simulink model "LKASampleSimulink"  (Simulink 9.1)
settings: Solver=ode1  StartTime=0.0  StopTime=inf  FixedStep=0.001  RelTol=1e-3
InitFcn:
  | load('LKAExampleVariable.mat')
values from neighbouring files (symbols this model uses):
  DataStoreNumPara = 0    [LKAExampleVariable.mat]
  headwayOffset = 3.7    [LKAExampleVariable.mat]
undefined symbols (not defined in the file or in its folder): azimuth_angle, BrStatus, elevation_angle, GroundTruth_Objects, heading, id, Lane_Car_Distance_Left, Lane_Car_Distance_Right, Lane_Class, Lane_Coefficient_C0, Lane_Coefficient_C1, Lane_Coefficient_C2, Lane_Coefficient_C3, Lane_Curvature, Lane_Distance, Lane_ID, LaneInfoPerception, range_bbox, range_center, shape, time, Timestamp, type, velocity, width
libraries: mpcadaslib x1
(part 2 of 2)

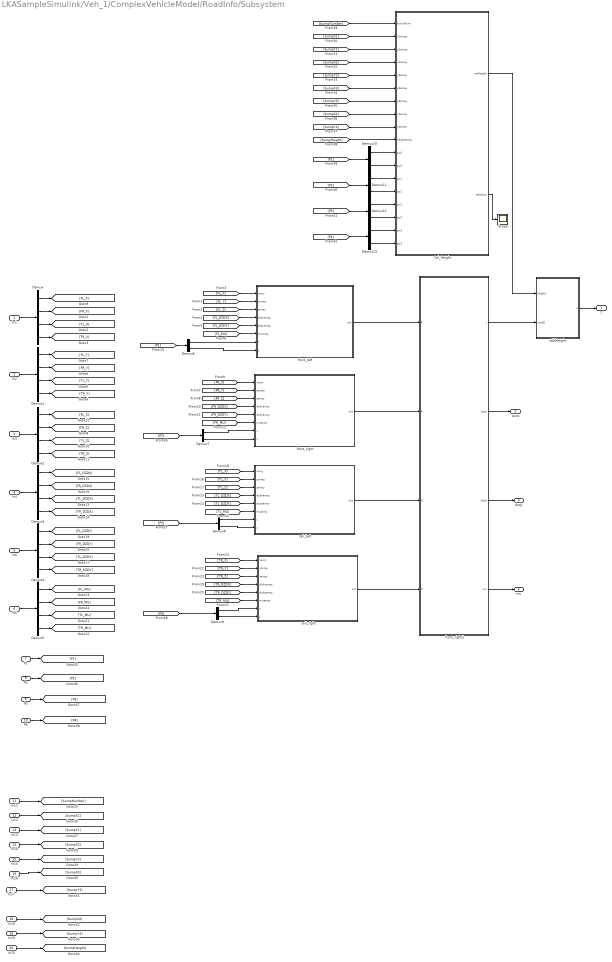
== system LKASampleSimulink/Veh_1/ComplexVehicleModel/RoadInfo/Subsystem ==
  In1 : Inport
  In2 : Inport  Port=2
  In3 : Inport  Port=3
  In4 : Inport  Port=4
  In6 : Inport  Port=5
  In5 : Inport  Port=6
  P1 : Inport  Port=7
  P2 : Inport  Port=8
  P3 : Inport  Port=9
  P4 : Inport  Port=10
  In11 : Inport  Port=11
  In12 : Inport  Port=12
  In13 : Inport  Port=13
  In14 : Inport  Port=14
  In15 : Inport  Port=15
  In16 : Inport  Port=16
  In17 : Inport  Port=17
  In18 : Inport  Port=18
  In19 : Inport  Port=19
  In20 : Inport  Port=20
  AddHeight : MATLAB Function  TreatAsAtomicUnit=on
  Cal_Height : MATLAB Function  TreatAsAtomicUnit=on
  Demux{,1..5} (6 alike) : Demux
  Demux{6..13} (8 alike) : Demux  Outputs=2
  Scope : Scope
  front_left : MATLAB Function  TreatAsAtomicUnit=on
  front_right : MATLAB Function  TreatAsAtomicUnit=on
  front_right1 : MATLAB Function  TreatAsAtomicUnit=on
  tail_left : MATLAB Function  TreatAsAtomicUnit=on
  tail_right : MATLAB Function  TreatAsAtomicUnit=on
  z : Outport  VectorParamsAs1DForOutWhenUnconnected=off
  dzdx : Outport  Port=2  VectorParamsAs1DForOutWhenUnconnected=off
  dzdy : Outport  Port=3  VectorParamsAs1DForOutWhenUnconnected=off
  mu : Outport  Port=4  VectorParamsAs1DForOutWhenUnconnected=off
  wires:
  Cal_Height/2(retValue) -> Scope/1
  AddHeight/1(z) -> z/1
  Cal_Height/1(retHeight) -> AddHeight/1(height)
  [bumpY3] -> Cal_Height/7(y3array)
  Demux11/1 -> Cal_Height/13(px1)
  [bumpHeight] -> Cal_Height/10(heightarray)
  [bumpX1] -> Cal_Height/2(x1array)
  Demux11/2 -> Cal_Height/14(py1)
  [bumpY1] -> Cal_Height/3(y1array)
  [P2] -> Demux11/1
  Demux10/1 -> Cal_Height/11(px0)
  [bumpX3] -> Cal_Height/6(x3array)
  [P3] -> Demux12/1
  Demux10/2 -> Cal_Height/12(py0)
  [bumpNumber] -> Cal_Height/1(bumsNum)
  Demux12/1 -> Cal_Height/15(px2)
  [P4] -> Demux13/1
  Demux12/2 -> Cal_Height/16(py2)
  [bumpY4] -> Cal_Height/9(y4array)
  [bumpX4] -> Cal_Height/8(x4array)
  [P1] -> Demux10/1
  [bumpX2] -> Cal_Height/4(x2array)
  Demux13/1 -> Cal_Height/17(px3)
  Demux13/2 -> Cal_Height/18(py3)
  [bumpY2] -> Cal_Height/5(y2array)
  [P4] -> Demux9/1
  [P3] -> Demux8/1
  [P2] -> Demux7/1
  [P1] -> Demux6/1
  In20/1 -> [bumpHeight]
  In19/1 -> [bumpY4]
  In18/1 -> [bumpX4]
  In17/1 -> [bumpY3]
  In16/1 -> [bumpX3]
  In15/1 -> [bumpY2]
  In14/1 -> [bumpX2]
  In13/1 -> [bumpY1]
  In12/1 -> [bumpX1]
  In11/1 -> [bumpNumber]
  In1/1 -> Demux/1
  Demux/1 -> [FL_X]
  Demux/2 -> [FR_X]
  Demux/3 -> [TL_X]
  Demux/4 -> [TR_X]
  Demux1/1 -> [FL_Y]
  Demux1/3 -> [TL_Y]
  Demux1/4 -> [TR_Y]
  Demux1/2 -> [FR_Y]
  In2/1 -> Demux1/1
  In3/1 -> Demux2/1
  Demux2/4 -> [TR_Z]
  Demux2/3 -> [TL_Z]
  Demux2/2 -> [FR_Z]
  Demux2/1 -> [FL_Z]
  Demux3/4 -> [TR_DZDX]
  In4/1 -> Demux3/1
  Demux3/3 -> [TL_DZDX]
  Demux3/1 -> [FL_DZDX]
  Demux3/2 -> [FR_DZDX]
  Demux4/2 -> [FR_DZDY]
  Demux4/4 -> [TR_DZDY]
  Demux4/1 -> [FL_DZDY]
  Demux4/3 -> [TL_DZDY]
  In6/1 -> Demux4/1
  Demux5/3 -> [TL_MU]
  Demux5/4 -> [TR_MU]
  Demux5/2 -> [FR_MU]
  Demux5/1 -> [FL_MU]
  In5/1 -> Demux5/1
  [FL_X] -> front_left/1(xarry)
  [FL_Y] -> front_left/2(yarray)
  [FL_MU] -> front_left/6(muarray)
  [FL_DZDY] -> front_left/5(dzdyarray)
  [FL_DZDX] -> front_left/4(dzdxarray)
  [FL_Z] -> front_left/3(zarray)
  [FR_X] -> front_right/1(xarry)
  [FR_Y] -> front_right/2(yarray)
  [FR_Z] -> front_right/3(zarray)
  [FR_DZDX] -> front_right/4(dzdxarray)
  [FR_DZDY] -> front_right/5(dzdyarray)
  [FR_MU] -> front_right/6(muarray)
  [TL_X] -> tail_left/1(xarry)
  [TL_Y] -> tail_left/2(yarray)
  [TL_Z] -> tail_left/3(zarray)
  [TL_DZDX] -> tail_left/4(dzdxarray)
  [TL_DZDY] -> tail_left/5(dzdyarray)
  [TL_MU] -> tail_left/6(muarray)
  [TR_X] -> tail_right/1(xarry)
  [TR_Y] -> tail_right/2(yarray)
  [TR_Z] -> tail_right/3(zarray)
  [TR_DZDX] -> tail_right/4(dzdxarray)
  [TR_DZDY] -> tail_right/5(dzdyarray)
  [TR_MU] -> tail_right/6(muarray)
  front_left/1(out) -> front_right1/1(fl)
  front_right/1(out) -> front_right1/2(fr)
  front_right1/1(z) -> AddHeight/2(roadZ)
  front_right1/2(dzdx) -> dzdx/1
  front_right1/3(dzdy) -> dzdy/1
  front_right1/4(mu) -> mu/1
  tail_left/1(out) -> front_right1/3(tl)
  tail_right/1(out) -> front_right1/4(tr)
  P1/1 -> [P1]
  Demux6/1 -> front_left/7(x)
  Demux6/2 -> front_left/8(y)
  P2/1 -> [P2]
  Demux7/1 -> front_right/7(x)
  Demux7/2 -> front_right/8(y)
  Demux8/1 -> tail_left/7(x)
  Demux8/2 -> tail_left/8(y)
  P3/1 -> [P3]
  Demux9/1 -> tail_right/7(x)
  Demux9/2 -> tail_right/8(y)
  P4/1 -> [P4]

== system LKASampleSimulink/Veh_1/ComplexVehicleModel/RoadInfo/Subsystem1 ==
  Rx_eo2ctc_coE_Refine : Inport
  Ry_eo2ctc_coE_Refine : Inport  Port=2
  front_right : MATLAB Function  TreatAsAtomicUnit=on
  P1 : Outport  VectorParamsAs1DForOutWhenUnconnected=off
  P2 : Outport  Port=2  VectorParamsAs1DForOutWhenUnconnected=off
  P3 : Outport  Port=3  VectorParamsAs1DForOutWhenUnconnected=off
  P4 : Outport  Port=4  VectorParamsAs1DForOutWhenUnconnected=off
  wires:
  Rx_eo2ctc_coE_Refine/1 -> front_right/1(array1)
  Ry_eo2ctc_coE_Refine/1 -> front_right/2(array2)
  front_right/2(p2) -> P2/1
  front_right/1(p1) -> P1/1
  front_right/3(p3) -> P3/1
  front_right/4(p4) -> P4/1

== system LKASampleSimulink/Veh_1/VehicleDataBus/GlobalVariableWrite/GlobalVariableSwitch ==
  value : Inport
  time : Inport  Port=2
  originalValue : Inport  Port=3
  originalTime : Inport  Port=4
  GlobalVariable0 : S-Function  FunctionName=BusWriter  Parameters='global.0','time@i,variable@d','0.01','0.0'  SFunctionDeploymentMode=off  EnableBusSupport=off
  Minus : Sum  Inputs=+-
  Switch : Switch  Criteria=u2 ~= 0  Threshold=1
  wires:
  Switch/1 -> GlobalVariable0/1
  originalTime/1 -> Switch/3
  time/1 -> Switch/1
  Minus/1 -> Switch/2
  originalValue/1 -> Minus/2
  value/1 -> Minus/1, GlobalVariable0/2

== system LKASampleSimulink/Veh_1/VehicleDataBus/GlobalVariableWrite/GlobalVariableSwitch1 ==
  value : Inport
  time : Inport  Port=2
  originalValue : Inport  Port=3
  originalTime : Inport  Port=4
  GlobalVariable1 : S-Function  FunctionName=BusWriter  Parameters='global.1','time@i,variable@d','0.01','0.0'  SFunctionDeploymentMode=off  EnableBusSupport=off
  Minus : Sum  Inputs=+-
  Switch : Switch  Criteria=u2 ~= 0  Threshold=1
  wires:
  Switch/1 -> GlobalVariable1/1
  originalTime/1 -> Switch/3
  time/1 -> Switch/1
  Minus/1 -> Switch/2
  originalValue/1 -> Minus/2
  value/1 -> Minus/1, GlobalVariable1/2

== system LKASampleSimulink/Veh_1/VehicleDataBus/GlobalVariableWrite/GlobalVariableSwitch2 ==
  value : Inport
  time : Inport  Port=2
  originalValue : Inport  Port=3
  originalTime : Inport  Port=4
  GlobalVariable2 : S-Function  FunctionName=BusWriter  Parameters='global.2','time@i,variable@d','0.01','0.0'  SFunctionDeploymentMode=off  EnableBusSupport=off
  Minus : Sum  Inputs=+-
  Switch : Switch  Criteria=u2 ~= 0  Threshold=1
  wires:
  Switch/1 -> GlobalVariable2/1
  originalTime/1 -> Switch/3
  time/1 -> Switch/1
  Minus/1 -> Switch/2
  originalValue/1 -> Minus/2
  value/1 -> Minus/1, GlobalVariable2/2

== system LKASampleSimulink/Veh_1/VehicleDataBus/GlobalVariableWrite/GlobalVariableSwitch3 ==
  value : Inport
  time : Inport  Port=2
  originalValue : Inport  Port=3
  originalTime : Inport  Port=4
  GlobalVariable3 : S-Function  FunctionName=BusWriter  Parameters='global.3','time@i,variable@d','0.01','0.0'  SFunctionDeploymentMode=off  EnableBusSupport=off
  Minus : Sum  Inputs=+-
  Switch : Switch  Criteria=u2 ~= 0  Threshold=1
  wires:
  Switch/1 -> GlobalVariable3/1
  originalTime/1 -> Switch/3
  time/1 -> Switch/1
  Minus/1 -> Switch/2
  originalValue/1 -> Minus/2
  value/1 -> Minus/1, GlobalVariable3/2

== system LKASampleSimulink/Veh_1/VehicleDataBus/GlobalVariableWrite/GlobalVariableSwitch4 ==
  value : Inport
  time : Inport  Port=2
  originalValue : Inport  Port=3
  originalTime : Inport  Port=4
  GlobalVariable4 : S-Function  FunctionName=BusWriter  Parameters='global.4','time@i,variable@d','0.01','0.0'  SFunctionDeploymentMode=off  EnableBusSupport=off
  Minus : Sum  Inputs=+-
  Switch : Switch  Criteria=u2 ~= 0  Threshold=1
  wires:
  Switch/1 -> GlobalVariable4/1
  originalTime/1 -> Switch/3
  time/1 -> Switch/1
  Minus/1 -> Switch/2
  originalValue/1 -> Minus/2
  value/1 -> Minus/1, GlobalVariable4/2

== system LKASampleSimulink/Veh_1/VehicleDataBus/GlobalVariableWrite/GlobalVariableSwitch5 ==
  value : Inport
  time : Inport  Port=2
  originalValue : Inport  Port=3
  originalTime : Inport  Port=4
  GlobalVariable5 : S-Function  FunctionName=BusWriter  Parameters='global.5','time@i,variable@d','0.01','0.0'  SFunctionDeploymentMode=off  EnableBusSupport=off
  Minus : Sum  Inputs=+-
  Switch : Switch  Criteria=u2 ~= 0  Threshold=1
  wires:
  Switch/1 -> GlobalVariable5/1
  originalTime/1 -> Switch/3
  time/1 -> Switch/1
  Minus/1 -> Switch/2
  originalValue/1 -> Minus/2
  value/1 -> Minus/1, GlobalVariable5/2

== system LKASampleSimulink/Veh_1/VehicleDataBus/GlobalVariableWrite/GlobalVariableSwitch6 ==
  value : Inport
  time : Inport  Port=2
  originalValue : Inport  Port=3
  originalTime : Inport  Port=4
  GlobalVariable6 : S-Function  FunctionName=BusWriter  Parameters='global.6','time@i,variable@d','0.01','0.0'  SFunctionDeploymentMode=off  EnableBusSupport=off
  Minus : Sum  Inputs=+-
  Switch : Switch  Criteria=u2 ~= 0  Threshold=1
  wires:
  Switch/1 -> GlobalVariable6/1
  originalTime/1 -> Switch/3
  time/1 -> Switch/1
  Minus/1 -> Switch/2
  originalValue/1 -> Minus/2
  value/1 -> Minus/1, GlobalVariable6/2

== system LKASampleSimulink/Veh_1/VehicleDataBus/GlobalVariableWrite/GlobalVariableSwitch7 ==
  value : Inport
  time : Inport  Port=2
  originalValue : Inport  Port=3
  originalTime : Inport  Port=4
  GlobalVariable7 : S-Function  FunctionName=BusWriter  Parameters='global.7','time@i,variable@d','0.01','0.0'  SFunctionDeploymentMode=off  EnableBusSupport=off
  Minus : Sum  Inputs=+-
  Switch : Switch  Criteria=u2 ~= 0  Threshold=1
  wires:
  Switch/1 -> GlobalVariable7/1
  originalTime/1 -> Switch/3
  time/1 -> Switch/1
  Minus/1 -> Switch/2
  originalValue/1 -> Minus/2
  value/1 -> Minus/1, GlobalVariable7/2

== system LKASampleSimulink/Veh_1/VehicleDataBus/GlobalVariableWrite/GlobalVariableSwitch8 ==
  value : Inport
  time : Inport  Port=2
  originalValue : Inport  Port=3
  originalTime : Inport  Port=4
  GlobalVariable8 : S-Function  FunctionName=BusWriter  Parameters='global.8','time@i,variable@d','0.01','0.0'  SFunctionDeploymentMode=off  EnableBusSupport=off
  Minus : Sum  Inputs=+-
  Switch : Switch  Criteria=u2 ~= 0  Threshold=1
  wires:
  Switch/1 -> GlobalVariable8/1
  originalTime/1 -> Switch/3
  time/1 -> Switch/1
  Minus/1 -> Switch/2
  originalValue/1 -> Minus/2
  value/1 -> Minus/1, GlobalVariable8/2

== system LKASampleSimulink/Veh_1/VehicleDataBus/GlobalVariableWrite/GlobalVariableSwitch9 ==
  value : Inport
  time : Inport  Port=2
  originalValue : Inport  Port=3
  originalTime : Inport  Port=4
  GlobalVariable9 : S-Function  FunctionName=BusWriter  Parameters='global.9','time@i,variable@d','0.01','0.0'  SFunctionDeploymentMode=off  EnableBusSupport=off
  Minus : Sum  Inputs=+-
  Switch : Switch  Criteria=u2 ~= 0  Threshold=1
  wires:
  Switch/1 -> GlobalVariable9/1
  originalTime/1 -> Switch/3
  time/1 -> Switch/1
  Minus/1 -> Switch/2
  originalValue/1 -> Minus/2
  value/1 -> Minus/1, GlobalVariable9/2

== system LKASampleSimulink/Veh_1/Algorithm/lane Following Controller/MPC Controller/InValueLimiters ==
  RelativeDistanceIn : Inport
  RelativeVelocityIn : Inport  Port=2
  LongitudinalVelocityIn : Inport  Port=3
  Constant1 : Constant  Value=200
  Constant2 : Constant  Value=0
  Saturation : Saturate  UpperLimit=100  LowerLimit=0.00001
  Switch1 : Switch  Criteria=u2 > Threshold  Threshold=1000
  Switch2 : Switch  Criteria=u2 > Threshold  Threshold=1000
  Relative distance : Outport
  Relative velocity : Outport  Port=2
  Longitudinal velocity : Outport  Port=3
  wires:
  RelativeVelocityIn/1 -> Switch2/3
  Constant2/1 -> Switch2/1
  Constant1/1 -> Switch1/1
  LongitudinalVelocityIn/1 -> Saturation/1
  RelativeDistanceIn/1 -> Switch1/2, Switch1/3, Switch2/2
  Switch2/1 -> Relative velocity/1
  Switch1/1 -> Relative distance/1
  Saturation/1 -> Longitudinal velocity/1

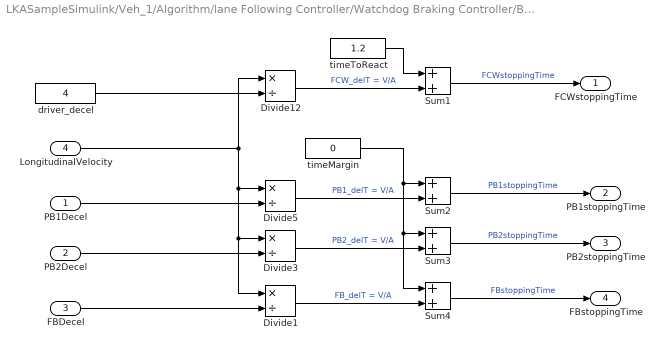
== system LKASampleSimulink/Veh_1/Algorithm/lane Following Controller/Watchdog Braking Controller/BrakeTimeCalculation ==
  PB1Decel : Inport
  PB2Decel : Inport  Port=2
  FBDecel : Inport  Port=3
  LongitudinalVelocity : Inport  Port=4
  Divide{1,3,5,12} (4 alike) : Product  Inputs=*/
  Sum{1..4} (4 alike) : Sum
  driver_decel : Constant  Value=4
  timeMargin : Constant  Value=0
  timeToReact : Constant  Value=1.2
  FCWstoppingTime : Outport
  PB1stoppingTime : Outport  Port=2
  PB2stoppingTime : Outport  Port=3
  FBstoppingTime : Outport  Port=4
  wires:
  Sum2/1 -> PB1stoppingTime/1  "PB1stoppingTime"
  timeMargin/1 -> Sum3/1, Sum4/1, Sum2/1
  Divide12/1 -> Sum1/2  "FCW_delT = V/A"
  LongitudinalVelocity/1 -> Divide3/1, Divide1/1, Divide5/1, Divide12/1
  PB2Decel/1 -> Divide3/2
  Divide1/1 -> Sum4/2  "FB_delT = V/A"
  Divide3/1 -> Sum3/2  "PB2_delT = V/A"
  Divide5/1 -> Sum2/2  "PB1_delT = V/A"
  timeToReact/1 -> Sum1/1
  FBDecel/1 -> Divide1/2
  driver_decel/1 -> Divide12/2
  PB1Decel/1 -> Divide5/2
  Sum4/1 -> FBstoppingTime/1  "FBstoppingTime"
  Sum3/1 -> PB2stoppingTime/1  "PB2stoppingTime"
  Sum1/1 -> FCWstoppingTime/1  "FCWstoppingTime"

== system LKASampleSimulink/Veh_1/Algorithm/lane Following Controller/Watchdog Braking Controller/BrakingLogic ==
  note: Input: relativeDistance, TTC, FCWtime, PB1time, PB2time, FBtime, longVelocity
      | Description: as time to collision gets shorter, request deceleration and signal the braking status. 4 Levels are identified warning, partial braking 1/2 and full braking.
      | Output: BrakeStatus, decel
  relativeDistance : Inport
  TTC : Inport  Port=2
  FCWtime : Inport  Port=3
  PB1time : Inport  Port=4
  PB2time : Inport  Port=5
  FBtime : Inport  Port=6
  longVelocity : Inport  Port=7
  BrakingLogic : Stateflow chart  TreatAsAtomicUnit=on
  RelationalOperator : RelationalOperator  Operator=<=  RndMeth=Simplest
  stopVelThreshold : Constant  Value=0.1
  BrakeStatus : Outport
  decel : Outport  Port=2
  wires:
  RelationalOperator/1 -> BrakingLogic/7(stop)
  relativeDistance/1 -> BrakingLogic/1(relativeDistance)
  BrakingLogic/2(decel) -> decel/1
  TTC/1 -> BrakingLogic/2(TTC)
  PB1time/1 -> BrakingLogic/4(PB1time)
  longVelocity/1 -> RelationalOperator/1
  FBtime/1 -> BrakingLogic/6(FBtime)
  FCWtime/1 -> BrakingLogic/3(FCWtime)
  BrakingLogic/1(BrakeStatus) -> BrakeStatus/1
  PB2time/1 -> BrakingLogic/5(PB2time)
  stopVelThreshold/1 -> RelationalOperator/2

== system LKASampleSimulink/Veh_1/Algorithm/lane Following Controller/Watchdog Braking Controller/TTCCalculation ==
  mioDistance : Inport
  mioVelocity : Inport  Port=2
  Abs : Abs
  Divide11 : Product  Inputs=**
  Divide3 : Product  Inputs=*/
  Saturation : Saturate  UpperLimit=100  LowerLimit=0.01
  Sign : Signum
  Sum : Sum  Inputs=+-
  const1 : Constant  Value=headwayOffset  SampleTime=-1
  TTC : Outport  VectorParamsAs1DForOutWhenUnconnected=off
  wires:
  mioVelocity/1 -> Sign/1, Abs/1
  mioDistance/1 -> Sum/1
  Divide3/1 -> Divide11/1  "TTC"
  const1/1 -> Sum/2
  Sum/1 -> Divide3/1  "headway"
  Abs/1 -> Saturation/1
  Saturation/1 -> Divide3/2
  Sign/1 -> Divide11/2
  Divide11/1 -> TTC/1

== matlab function Veh_1/ComplexVehicleModel/RoadInfo/Subsystem/front_right ==
  data: out output double; xarry input double; yarray input double; zarray input double; dzdxarray input double; dzdyarray input double; muarray input double; x input double; y input double
function out  = fcn(xarry,yarray,zarray,dzdxarray,dzdyarray,muarray,x,y)
[x1,y1,x2,y2,x3,y3,x4,y4] = fcn_getpoint(xarry,yarray);
data_array = fcn_getdata(zarray,dzdxarray, dzdyarray,muarray);

zero = 0.001;
if ( abs(y2-y1) > zero )
   angle = 2*pi -  atan2(y2-y1,x2-x1);
   sin_angle = sin(angle);
   cos_angle = cos(angle);
   [x1,y1] = fcn_convert(x1,y1,x1,y1,sin_angle,cos_angle);
   [x2,y2] = fcn_convert(x1,y1,x2,y2,sin_angle,cos_angle);
   [x3,y3] = fcn_convert(x1,y1,x3,y3,sin_angle,cos_angle);
   [x4,y4] = fcn_convert(x1,y1,x4,y4,sin_angle,cos_angle);
   [x,y] = fcn_convert(x1,y1,x,y,sin_angle,cos_angle);
end

axle_x_left  = min(x1,x2);
axle_x_right = max(x1,x2);
axle_y_up    = max(y2,y3);
axle_y_down  = min(y2,y3);

% after rotota
% p1  p2
%
% p3 p4
z = 0;
dzdx = 0;
dzdy = 0;
mu = 0;
if ( x > axle_x_left ) && ( x < axle_x_right ) && ( y > axle_y_down ) && ( y < axle_y_up )
    xx1 = x3;
    xx2 = x4;
    yy1 = y3;
    yy2 = y1;
    matrix_left = [xx2-x  x-xx1];
    matrix_right = [ yy2 - y; y-yy1 ];
    delta = (xx2-xx1)*(yy2-yy1);
    delta = 1.0/delta;
    [z, dzdx, dzdy, mu] = fcn_cal(matrix_left,matrix_right,delta,data_array);
else
    if ( y >= axle_y_up ) 
        [z, dzdx, dzdy, mu] = fcn_cal_getmax(data_array(1,:),data_array(2,:));
    end
    if ( y <= axle_y_down )
        [z, dzdx, dzdy, mu] = fcn_cal_getmax(data_array(3,:),data_array(4,:));
    end
    if ( x >= axle_x_right )
        [z, dzdx, dzdy, mu] = fcn_cal_getmax(data_array(2,:),data_array(4,:));
    end
    if ( x <= axle_x_left )
        [z, dzdx, dzdy, mu] = fcn_cal_getmax(data_array(1,:),data_array(3,:));
    end
end

out = [z dzdx dzdy mu];
end

function [xxx,yyy] = fcn_convert(x0,y0,x1,y1,sin_agnle,cos_angle)
    xxx = (x1-x0)*cos_angle - (y1-y0)*sin_agnle + x0;
    yyy = (x1-x0)*sin_agnle + (y1-y0)*cos_angle + y0;
end

function [x1,y1,x2,y2,x3,y3,x4,y4] = fcn_getpoint(xarry,yarray)
    x1 = xarry(1);
    x2 = xarry(2);
    x3 = xarry(3);
    x4 = xarry(4);
    y1 = yarray(1);
    y2 = yarray(2);
    y3 = yarray(3);
    y4 = yarray(4);
end

function ret = fcn_getdata(zarray,dzdxarray, dzdyarray,muarray)
    ret = [ 
        zarray(1),dzdxarray(1),dzdyarray(1),muarray(1);
        zarray(2),dzdxarray(2),dzdyarray(2),muarray(2);
        zarray(3),dzdxarray(3),dzdyarray(3),muarray(3);
        zarray(4),dzdxarray(4),dzdyarray(4),muarray(4);
    ];
end

function [z,dzdx,dzdy,mu] = fcn_cal(matrix_left,matrix_right , delta, data_array)
%matrix_z = [z3, z1; z4 , z2]
%value = [xx2-x  x-xx1] * matrix * [ yy2 - y; y-yy1 ]  * d1
    array_z = data_array(:,1);
    array_dzdx = data_array(:,2);
    array_dzdy = data_array(:,3);
    array_mu = data_array(:,4);
    z = matrix_left * [array_z(3), array_z(1); array_z(4),array_z(2)] * matrix_right  * delta;
    dzdx = matrix_left * [array_dzdx(3), array_dzdx(1); array_dzdx(4),array_dzdx(2)] * matrix_right  * delta;
    dzdy = matrix_left * [array_dzdy(3), array_dzdy(1); array_dzdy(4),array_dzdy(2)] * matrix_right  * delta;
    mu = matrix_left * [array_mu(3), array_mu(1); array_mu(4),array_mu(2)] * matrix_right  * delta;
end

function [z,dzdx,dzdy,mu] = fcn_cal_getmax(data1,data2)
    z = max(data1(1),data2(1));
    dzdx = max(data1(2),data2(2));
    dzdy = max(data1(3),data2(3));
    mu = max(data1(4),data2(4));
end

== matlab function Veh_1/ComplexVehicleModel/RoadInfo/Subsystem/front_left ==
  data: out output double; xarry input double; yarray input double; zarray input double; dzdxarray input double; dzdyarray input double; muarray input double; x input double; y input double
function out  = fcn(xarry,yarray,zarray,dzdxarray,dzdyarray,muarray,x,y)
[x1,y1,x2,y2,x3,y3,x4,y4] = fcn_getpoint(xarry,yarray);
data_array = fcn_getdata(zarray,dzdxarray, dzdyarray,muarray);

zero = 0.001;
if ( abs(y2-y1) > zero )
   angle = 2*pi -  atan2(y2-y1,x2-x1);
   sin_angle = sin(angle);
   cos_angle = cos(angle);
   [x1,y1] = fcn_convert(x1,y1,x1,y1,sin_angle,cos_angle);
   [x2,y2] = fcn_convert(x1,y1,x2,y2,sin_angle,cos_angle);
   [x3,y3] = fcn_convert(x1,y1,x3,y3,sin_angle,cos_angle);
   [x4,y4] = fcn_convert(x1,y1,x4,y4,sin_angle,cos_angle);
   [x,y] = fcn_convert(x1,y1,x,y,sin_angle,cos_angle);
end

axle_x_left  = min(x1,x2);
axle_x_right = max(x1,x2);
axle_y_up    = max(y2,y3);
axle_y_down  = min(y2,y3);

% after rotota
% p1  p2
%
% p3 p4
z = 0;
dzdx = 0;
dzdy = 0;
mu = 0;
if ( x > axle_x_left ) && ( x < axle_x_right ) && ( y > axle_y_down ) && ( y < axle_y_up )
    xx1 = x3;
    xx2 = x4;
    yy1 = y3;
    yy2 = y1;
    matrix_left = [xx2-x  x-xx1];
    matrix_right = [ yy2 - y; y-yy1 ];
    delta = (xx2-xx1)*(yy2-yy1);
    delta = 1.0/delta;
    [z, dzdx, dzdy, mu] = fcn_cal(matrix_left,matrix_right,delta,data_array);
else
    if ( y >= axle_y_up ) 
        [z, dzdx, dzdy, mu] = fcn_cal_getmax(data_array(1,:),data_array(2,:));
    end
    if ( y <= axle_y_down )
        [z, dzdx, dzdy, mu] = fcn_cal_getmax(data_array(3,:),data_array(4,:));
    end
    if ( x >= axle_x_right )
        [z, dzdx, dzdy, mu] = fcn_cal_getmax(data_array(2,:),data_array(4,:));
    end
    if ( x <= axle_x_left )
        [z, dzdx, dzdy, mu] = fcn_cal_getmax(data_array(1,:),data_array(3,:));
    end
end

out = [z dzdx dzdy mu];
end

function [xxx,yyy] = fcn_convert(x0,y0,x1,y1,sin_agnle,cos_angle)
    xxx = (x1-x0)*cos_angle - (y1-y0)*sin_agnle + x0;
    yyy = (x1-x0)*sin_agnle + (y1-y0)*cos_angle + y0;
end

function [x1,y1,x2,y2,x3,y3,x4,y4] = fcn_getpoint(xarry,yarray)
    x1 = xarry(1);
    x2 = xarry(2);
    x3 = xarry(3);
    x4 = xarry(4);
    y1 = yarray(1);
    y2 = yarray(2);
    y3 = yarray(3);
    y4 = yarray(4);
end

function ret = fcn_getdata(zarray,dzdxarray, dzdyarray,muarray)
    ret = [ 
        zarray(1),dzdxarray(1),dzdyarray(1),muarray(1);
        zarray(2),dzdxarray(2),dzdyarray(2),muarray(2);
        zarray(3),dzdxarray(3),dzdyarray(3),muarray(3);
        zarray(4),dzdxarray(4),dzdyarray(4),muarray(4);
    ];
end

function [z,dzdx,dzdy,mu] = fcn_cal(matrix_left,matrix_right , delta, data_array)
%matrix_z = [z3, z1; z4 , z2]
%value = [xx2-x  x-xx1] * matrix * [ yy2 - y; y-yy1 ]  * d1
    array_z = data_array(:,1);
    array_dzdx = data_array(:,2);
    array_dzdy = data_array(:,3);
    array_mu = data_array(:,4);
    z = matrix_left * [array_z(3), array_z(1); array_z(4),array_z(2)] * matrix_right  * delta;
    dzdx = matrix_left * [array_dzdx(3), array_dzdx(1); array_dzdx(4),array_dzdx(2)] * matrix_right  * delta;
    dzdy = matrix_left * [array_dzdy(3), array_dzdy(1); array_dzdy(4),array_dzdy(2)] * matrix_right  * delta;
    mu = matrix_left * [array_mu(3), array_mu(1); array_mu(4),array_mu(2)] * matrix_right  * delta;
end

function [z,dzdx,dzdy,mu] = fcn_cal_getmax(data1,data2)
    z = max(data1(1),data2(1));
    dzdx = max(data1(2),data2(2));
    dzdy = max(data1(3),data2(3));
    mu = max(data1(4),data2(4));
end

== matlab function Veh_1/ComplexVehicleModel/RoadInfo/Subsystem/tail_left ==
  data: out output double; xarry input double; yarray input double; zarray input double; dzdxarray input double; dzdyarray input double; muarray input double; x input double; y input double
function out  = fcn(xarry,yarray,zarray,dzdxarray,dzdyarray,muarray,x,y)
[x1,y1,x2,y2,x3,y3,x4,y4] = fcn_getpoint(xarry,yarray);
data_array = fcn_getdata(zarray,dzdxarray, dzdyarray,muarray);

zero = 0.001;
if ( abs(y2-y1) > zero )
   angle = 2*pi -  atan2(y2-y1,x2-x1);
   sin_angle = sin(angle);
   cos_angle = cos(angle);
   [x1,y1] = fcn_convert(x1,y1,x1,y1,sin_angle,cos_angle);
   [x2,y2] = fcn_convert(x1,y1,x2,y2,sin_angle,cos_angle);
   [x3,y3] = fcn_convert(x1,y1,x3,y3,sin_angle,cos_angle);
   [x4,y4] = fcn_convert(x1,y1,x4,y4,sin_angle,cos_angle);
   [x,y] = fcn_convert(x1,y1,x,y,sin_angle,cos_angle);
end

axle_x_left  = min(x1,x2);
axle_x_right = max(x1,x2);
axle_y_up    = max(y2,y3);
axle_y_down  = min(y2,y3);

% after rotota
% p1  p2
%
% p3 p4
z = 0;
dzdx = 0;
dzdy = 0;
mu = 0;
if ( x > axle_x_left ) && ( x < axle_x_right ) && ( y > axle_y_down ) && ( y < axle_y_up )
    xx1 = x3;
    xx2 = x4;
    yy1 = y3;
    yy2 = y1;
    matrix_left = [xx2-x  x-xx1];
    matrix_right = [ yy2 - y; y-yy1 ];
    delta = (xx2-xx1)*(yy2-yy1);
    delta = 1.0/delta;
    [z, dzdx, dzdy, mu] = fcn_cal(matrix_left,matrix_right,delta,data_array);
else
    if ( y >= axle_y_up ) 
        [z, dzdx, dzdy, mu] = fcn_cal_getmax(data_array(1,:),data_array(2,:));
    end
    if ( y <= axle_y_down )
        [z, dzdx, dzdy, mu] = fcn_cal_getmax(data_array(3,:),data_array(4,:));
    end
    if ( x >= axle_x_right )
        [z, dzdx, dzdy, mu] = fcn_cal_getmax(data_array(2,:),data_array(4,:));
    end
    if ( x <= axle_x_left )
        [z, dzdx, dzdy, mu] = fcn_cal_getmax(data_array(1,:),data_array(3,:));
    end
end

out = [z dzdx dzdy mu];
end

function [xxx,yyy] = fcn_convert(x0,y0,x1,y1,sin_agnle,cos_angle)
    xxx = (x1-x0)*cos_angle - (y1-y0)*sin_agnle + x0;
    yyy = (x1-x0)*sin_agnle + (y1-y0)*cos_angle + y0;
end

function [x1,y1,x2,y2,x3,y3,x4,y4] = fcn_getpoint(xarry,yarray)
    x1 = xarry(1);
    x2 = xarry(2);
    x3 = xarry(3);
    x4 = xarry(4);
    y1 = yarray(1);
    y2 = yarray(2);
    y3 = yarray(3);
    y4 = yarray(4);
end

function ret = fcn_getdata(zarray,dzdxarray, dzdyarray,muarray)
    ret = [ 
        zarray(1),dzdxarray(1),dzdyarray(1),muarray(1);
        zarray(2),dzdxarray(2),dzdyarray(2),muarray(2);
        zarray(3),dzdxarray(3),dzdyarray(3),muarray(3);
        zarray(4),dzdxarray(4),dzdyarray(4),muarray(4);
    ];
end

function [z,dzdx,dzdy,mu] = fcn_cal(matrix_left,matrix_right , delta, data_array)
%matrix_z = [z3, z1; z4 , z2]
%value = [xx2-x  x-xx1] * matrix * [ yy2 - y; y-yy1 ]  * d1
    array_z = data_array(:,1);
    array_dzdx = data_array(:,2);
    array_dzdy = data_array(:,3);
    array_mu = data_array(:,4);
    z = matrix_left * [array_z(3), array_z(1); array_z(4),array_z(2)] * matrix_right  * delta;
    dzdx = matrix_left * [array_dzdx(3), array_dzdx(1); array_dzdx(4),array_dzdx(2)] * matrix_right  * delta;
    dzdy = matrix_left * [array_dzdy(3), array_dzdy(1); array_dzdy(4),array_dzdy(2)] * matrix_right  * delta;
    mu = matrix_left * [array_mu(3), array_mu(1); array_mu(4),array_mu(2)] * matrix_right  * delta;
end

function [z,dzdx,dzdy,mu] = fcn_cal_getmax(data1,data2)
    z = max(data1(1),data2(1));
    dzdx = max(data1(2),data2(2));
    dzdy = max(data1(3),data2(3));
    mu = max(data1(4),data2(4));
end

== matlab function Veh_1/ComplexVehicleModel/RoadInfo/Subsystem/tail_right ==
  data: out output double; xarry input double; yarray input double; zarray input double; dzdxarray input double; dzdyarray input double; muarray input double; x input double; y input double
function out  = fcn(xarry,yarray,zarray,dzdxarray,dzdyarray,muarray,x,y)
[x1,y1,x2,y2,x3,y3,x4,y4] = fcn_getpoint(xarry,yarray);
data_array = fcn_getdata(zarray,dzdxarray, dzdyarray,muarray);

zero = 0.001;
if ( abs(y2-y1) > zero )
   angle = 2*pi -  atan2(y2-y1,x2-x1);
   sin_angle = sin(angle);
   cos_angle = cos(angle);
   [x1,y1] = fcn_convert(x1,y1,x1,y1,sin_angle,cos_angle);
   [x2,y2] = fcn_convert(x1,y1,x2,y2,sin_angle,cos_angle);
   [x3,y3] = fcn_convert(x1,y1,x3,y3,sin_angle,cos_angle);
   [x4,y4] = fcn_convert(x1,y1,x4,y4,sin_angle,cos_angle);
   [x,y] = fcn_convert(x1,y1,x,y,sin_angle,cos_angle);
end

axle_x_left  = min(x1,x2);
axle_x_right = max(x1,x2);
axle_y_up    = max(y2,y3);
axle_y_down  = min(y2,y3);

% after rotota
% p1  p2
%
% p3 p4
z = 0;
dzdx = 0;
dzdy = 0;
mu = 0;
if ( x > axle_x_left ) && ( x < axle_x_right ) && ( y > axle_y_down ) && ( y < axle_y_up )
    xx1 = x3;
    xx2 = x4;
    yy1 = y3;
    yy2 = y1;
    matrix_left = [xx2-x  x-xx1];
    matrix_right = [ yy2 - y; y-yy1 ];
    delta = (xx2-xx1)*(yy2-yy1);
    delta = 1.0/delta;
    [z, dzdx, dzdy, mu] = fcn_cal(matrix_left,matrix_right,delta,data_array);
else
    if ( y >= axle_y_up ) 
        [z, dzdx, dzdy, mu] = fcn_cal_getmax(data_array(1,:),data_array(2,:));
    end
    if ( y <= axle_y_down )
        [z, dzdx, dzdy, mu] = fcn_cal_getmax(data_array(3,:),data_array(4,:));
    end
    if ( x >= axle_x_right )
        [z, dzdx, dzdy, mu] = fcn_cal_getmax(data_array(2,:),data_array(4,:));
    end
    if ( x <= axle_x_left )
        [z, dzdx, dzdy, mu] = fcn_cal_getmax(data_array(1,:),data_array(3,:));
    end
end

out = [z dzdx dzdy mu];
end

function [xxx,yyy] = fcn_convert(x0,y0,x1,y1,sin_agnle,cos_angle)
    xxx = (x1-x0)*cos_angle - (y1-y0)*sin_agnle + x0;
    yyy = (x1-x0)*sin_agnle + (y1-y0)*cos_angle + y0;
end

function [x1,y1,x2,y2,x3,y3,x4,y4] = fcn_getpoint(xarry,yarray)
    x1 = xarry(1);
    x2 = xarry(2);
    x3 = xarry(3);
    x4 = xarry(4);
    y1 = yarray(1);
    y2 = yarray(2);
    y3 = yarray(3);
    y4 = yarray(4);
end

function ret = fcn_getdata(zarray,dzdxarray, dzdyarray,muarray)
    ret = [ 
        zarray(1),dzdxarray(1),dzdyarray(1),muarray(1);
        zarray(2),dzdxarray(2),dzdyarray(2),muarray(2);
        zarray(3),dzdxarray(3),dzdyarray(3),muarray(3);
        zarray(4),dzdxarray(4),dzdyarray(4),muarray(4);
    ];
end

function [z,dzdx,dzdy,mu] = fcn_cal(matrix_left,matrix_right , delta, data_array)
%matrix_z = [z3, z1; z4 , z2]
%value = [xx2-x  x-xx1] * matrix * [ yy2 - y; y-yy1 ]  * d1
    array_z = data_array(:,1);
    array_dzdx = data_array(:,2);
    array_dzdy = data_array(:,3);
    array_mu = data_array(:,4);
    z = matrix_left * [array_z(3), array_z(1); array_z(4),array_z(2)] * matrix_right  * delta;
    dzdx = matrix_left * [array_dzdx(3), array_dzdx(1); array_dzdx(4),array_dzdx(2)] * matrix_right  * delta;
    dzdy = matrix_left * [array_dzdy(3), array_dzdy(1); array_dzdy(4),array_dzdy(2)] * matrix_right  * delta;
    mu = matrix_left * [array_mu(3), array_mu(1); array_mu(4),array_mu(2)] * matrix_right  * delta;
end

function [z,dzdx,dzdy,mu] = fcn_cal_getmax(data1,data2)
    z = max(data1(1),data2(1));
    dzdx = max(data1(2),data2(2));
    dzdy = max(data1(3),data2(3));
    mu = max(data1(4),data2(4));
end

== matlab function Veh_1/ComplexVehicleModel/RoadInfo/Subsystem/front_right1 ==
  data: z output double; fl input double; fr input double; tl input double; tr input double; dzdx output double; dzdy output double; mu output double
function [z,dzdx,dzdy,mu]  = fcn(fl,fr,tl,tr)
    z =  [fl(1),fr(1),tl(1),tr(1)];
    dzdx = [fl(2),fr(2),tl(2),tr(2)];
    dzdy = [fl(3),fr(3),tl(3),tr(3)];
    mu =   [fl(4),fr(4),tl(4),tr(4)];
end

== matlab function Veh_1/ComplexVehicleModel/RoadInfo/Subsystem1/front_right ==
  data: p1 output double; array1 input double; array2 input double; p2 output double; p3 output double; p4 output double
function [p1,p2,p3,p4]  = fcn(array1,array2)
    p1 = [array1(1),array2(1)];
    p2 = [array1(2),array2(2)];
    p3 = [array1(3),array2(3)];
    p4 = [array1(4),array2(4)];
end

== matlab function Veh_1/ComplexVehicleModel/RoadInfo/Subsystem/Cal_Height ==
  data: retHeight output double; bumsNum input double; x1array input double; y1array input double; x2array input double; y2array input double; x3array input double; y3array input double; x4array input double; y4array input double; heightarray input double; px0 input double; py0 input double; px1 input double; py1 input double; px2 input double; py2 input double; px3 input double; py3 input double; retValue output double
function [retHeight,retValue]   = fcn(bumsNum,x1array,y1array,x2array,y2array,x3array,y3array,x4array,y4array,heightarray,px0,py0,px1,py1,px2,py2,px3,py3)
h0 = 0.0;
h1 = 0.0;
h2 = 0.0;
h3 = 0.0;
value0 = 0;
value1 = 0;
value2 = 0;
value3 = 0;
for index = 1:bumsNum+1
     v = fcn_in_sqar(x1array(index),y1array(index),x2array(index),y2array(index),x3array(index),y3array(index),x4array(index),y4array(index),px0,py0);
     if (v > 0)
         value0 = 1;
         h0 =  heightarray(index);
         break;
     end
end
for index = 1:bumsNum+1
     v = fcn_in_sqar(x1array(index),y1array(index),x2array(index),y2array(index),x3array(index),y3array(index),x4array(index),y4array(index),px1,py1);
     if (v > 0)
         value1 = 1;
         h1 =  heightarray(index);
         break;
     end
end

for index = 1:bumsNum+1
     v = fcn_in_sqar(x1array(index),y1array(index),x2array(index),y2array(index),x3array(index),y3array(index),x4array(index),y4array(index),px2,py2);
     if (v > 0)
         value2 = 1;
         h2 =  heightarray(index);
         break;
     end
end

for index = 1:bumsNum+1
     v = fcn_in_sqar(x1array(index),y1array(index),x2array(index),y2array(index),x3array(index),y3array(index),x4array(index),y4array(index),px3,py3);
     if (v > 0)
         value3 = 1;
         h3 =  heightarray(index);
         break;
     end
end
retHeight = [h0,h1,h2,h3];
retValue = [value0,value1,value2,value3];
end


function ret = fcn_in_sqar(x1,y1,x2,y2,x3,y3,x4,y4,x,y)
    ret = 0;
    a = (x2-x1)*(y-y1)-(y2-y1)*(x-x1);
    b = (x3-x2)*(y-y2)-(y3-y2)*(x-x2);
    c = (x4-x3)*(y-y3)-(y4-y3)*(x-x3);
    d = (x1-x4)*(y-y4)-(y1-y4)*(x-x4);
    if (a>=0&&b>=0&&c>=0&&d>=0)
        ret = 1;
    end
    if (a<=0&&b<=0&&c<=0&&d<=0)
        ret = 1;
    end
end

== matlab function Veh_1/ComplexVehicleModel/RoadInfo/Subsystem/AddHeight ==
  data: z output double; height input double; roadZ input double
function z  = fcn(height,roadZ)
    z =  [roadZ(1)+height(1),roadZ(2)+height(2),roadZ(3)+height(3),roadZ(4)+height(4)];
end

== matlab function Veh_1/Algorithm/ControlSignalFilter/MATLAB Function ==
  data: driver input double; valid output double; algoThrottle input double; algoBrake input double; algoSteer input double; algoMode input double; algoGear input double; throttle output double; brake output double; steer output double; mode output double; gear output double
function [valid,throttle,brake,steer,mode,gear] = fcn(driver,algoThrottle,algoBrake,algoSteer,algoMode,algoGear)
valid = driver(1) + algoThrottle(2) + algoBrake(2) + algoSteer(2) + algoMode(2) + algoGear(2);
if valid > 0
    valid = 1;
end

throttle = fcnValidData(driver(2),algoThrottle(3),algoThrottle(2));
brake = fcnValidData(driver(3),algoBrake(3),algoBrake(2));
steer = fcnValidData(driver(4),algoSteer(3),algoSteer(2));
mode = fcnValidData(driver(5),algoMode(3),algoMode(2));
gear = fcnValidData(driver(6),algoGear(3),algoGear(2));

end

function out = fcnValidData(data1,data2,valid)
    if valid > 0.5
        out = data2;
    else
        out = data1;
    end
end

== matlab function Veh_1/ComplexVehicleModel/RoadInfo/MATLAB Function ==
  data: fl input double; tire_x output double; fr input double; rl input double; rr input double; tire_y output double; tire_z output double
function [tire_x,tire_y,tire_z] = fcn(fl,fr,rl,rr)

tire_x = [fl(11),fr(11),rl(11),rr(11)];
tire_y = [fl(12),fr(12),rl(12),rr(12)];
tire_z = [fl(13),fr(13),rl(13),rr(13)];

== matlab function Veh_1/ComplexVehicleModel/RoadInfo/MATLAB Function1 ==
  data: t input double; outz output double; z input double; dzdx input double; dzdy input double; mu input double; tirez input double; outdzdx output double; outdzdy output double; outmu output double
function [outz,outdzdx,outdzdy,outmu] = fcn(t,z,dzdx,dzdy,mu,tirez)
%#codegen
outz = tirez;
outdzdx = [0,0,0,0];
outdzdy = [0,0,0,0];
outmu = [0.75,0.75,0.75,0.75];
if t > 0.001
    outz = z;
    outdzdx = dzdx;
    outdzdy = dzdy;
    outmu = mu;
end

== matlab function Veh_1/VehicleDataBus/MATLAB Function ==
  data: u input double; head output double; c_x output double; c_y output double; c_z output double; yaw output double; pitch output double; roll output double; rot_spd output double; f_x output double; f_y output double; f_z output double; g_x output double; g_y output double; g_z output double
function [head,c_x,c_y,c_z,yaw,pitch,roll,rot_spd,f_x,f_y,f_z,g_x,g_y,g_z] = fcn(u)
head = [u(1),u(2),u(3),u(4),u(5)];
start = 6;
c_x =   [u(start),u(start+13),u(start+26),u(start+39)];
start = 7;
c_y =   [u(start),u(start+13),u(start+26),u(start+39)];
start = 8;
c_z =   [u(start),u(start+13),u(start+26),u(start+39)];
start = 9;
yaw =   [u(start),u(start+13),u(start+26),u(start+39)];
start = 10;
pitch = [u(start),u(start+13),u(start+26),u(start+39)];
start = 11;
roll =  [u(start),u(start+13),u(start+26),u(start+39)];
start = 12;
rot_spd =  [u(start),u(start+13),u(start+26),u(start+39)];
start = 13;
f_x =  [u(start),u(start+13),u(start+26),u(start+39)];
start = 14;
f_y =  [u(start),u(start+13),u(start+26),u(start+39)];
start = 15;
f_z =  [u(start),u(start+13),u(start+26),u(start+39)];
start = 16;
g_x =  [u(start),u(start+13),u(start+26),u(start+39)];
start = 17;
g_y =  [u(start),u(start+13),u(start+26),u(start+39)];
start = 18;
g_z =  [u(start),u(start+13),u(start+26),u(start+39)];

== matlab function Veh_1/ComplexVehicleModel/MATLAB Function1 ==
  data: u input double; ego output double; egoextra output double
function [ego,egoextra] = fcn(u)

ego = [u(2),u(3),u(4),u(5),u(6),u(7),u(8)];
egoextra = [u(8),u(9),u(10),u(11),u(12),u(13),u(14),u(15),u(16),u(17),u(18),u(19)];

== matlab function Veh_1/ComplexVehicleModel/MATLAB Function2 ==
  data: driverControl input double; throttle output double; dynamicControl input double; brake output double; steer output double; mode output double
function [throttle,brake,steer,mode] = fcn(driverControl,dynamicControl)
%#codegen
if driverControl(1) > 0.5
    throttle = driverControl(2);
    brake = driverControl(3)* 1e6;
    steer = driverControl(4) * 0.0174;
    mode = driverControl(5);
else
    throttle = dynamicControl(3);
    brake = dynamicControl(4);
    steer = dynamicControl(5);
    mode = dynamicControl(2);
end

if mode > 0.5
   mode = 1 ;
end

== matlab function Veh_1/Algorithm/Lane Following Decision Logic/MATLAB Function ==
  data: data_t input double; curvature output double; curvature_devi output double; headingAngle output double; latOffset output double; leftDis input double; rightDis input double; curv input double; C0 input double; C1 input double; C2 input double; C3 input double
function [curvature,curvature_devi, headingAngle,latOffset]  = fcn (data_t, leftDis,rightDis,curv,C0,C1,C2,C3)

leftID = 2;
if data_t > 0
    curvature = curv(leftID);
    curvature_devi = 0;
    headingAngle = atan(C1(2));
    if abs(headingAngle) < 0.01
        headingAngle = 0;
    end
    latOffset = leftDis(2)-0.85;
else
    curvature = 0;
    curvature_devi = 0;
    headingAngle = 0;
    latOffset = 0;
end
end

== stateflow chart Veh_1/Algorithm/lane Following Controller/Watchdog Braking Controller/BrakingLogic/BrakingLogic ==
  state Default
    entry:
    BrakeStatus = BrStatus.NoBrake;
    decel = Default_decel;
  state FCW
    entry:
    BrakeStatus = BrStatus.NoBrake;
    decel = Default_decel;
  state Partial_Braking1
    entry:
    BrakeStatus = BrStatus.PB1Brake;
    decel = PB1_decel;
  state Partial_Braking2
    entry:
    BrakeStatus =BrStatus.PB2Brake;
    decel = PB2_decel;
  state Full_Braking
    entry:
    BrakeStatus = BrStatus.FBrake;
    decel = FB_decel;
  (default) -> Default
  Default -> (junction 236) [order 2]
  (junction 236) -> Full_Braking : [relativeDistance < default_spacing]
  (junction 237) -> Default
  Full_Braking -> (junction 237) : [stop && TTC>double(0) && relativeDistance > default_spacing ]
  (junction 238) -> Default
  (junction 241) -> (junction 238) : [stop]
  (junction 239) -> Default
  (junction 240) -> (junction 239) : [stop]
  Default -> FCW [order 1] : [(abs(TTC)<FCWtime) && TTC<double(0)]
  FCW -> Default [order 2] : [abs(TTC)>=TimeFactor*FCWtime]
  FCW -> Partial_Braking1 [order 1] : [(abs(TTC) < PB1time) && TTC<double(0)]
  Partial_Braking1 -> (junction 240) [order 2]
  Partial_Braking1 -> Partial_Braking2 [order 1] : [(abs(TTC) < PB2time) && TTC<double(0)]
  Partial_Braking2 -> (junction 241) [order 2]
  Partial_Braking2 -> Full_Braking [order 1] : [(abs(TTC) < FBtime) && TTC<double(0)]
  data: relativeDistance input double; TTC input double; FCWtime input double; PB1time input double; PB2time input double; FBtime input double; BrakeStatus output uint8; decel output double; stop input boolean; FB_decel constant double =FB_decel; PB2_decel constant double =PB2_decel; Default_decel constant double =Default_decel; TimeFactor constant double =TimeFactor; PB1_decel constant double =PB1_decel; default_spacing constant double =default_spacing

== matlab function Veh_1/Algorithm/Lane Following Decision Logic/Find Leader Car ==
  data: EGOX input double; RelatedDistance output double; EGOY input double; EGOV input double; EGOYAW input double; time input double; width input double; ids input double; types input double; shapes input double; range_centers input double; range_bboxs input double; azimuth_angles input double; elevation_angles input double; velocitys input double; headings input double; RelatedSpeed output double
function [RelatedDistance, RelatedSpeed]  = DetectionConcatenation(EGOX,EGOY,EGOV, EGOYAW, time, width, ids, types, shapes, range_centers, range_bboxs, azimuth_angles, elevation_angles, velocitys, headings)


% This function finds the lead car: a car in front of the ego car that
% satisfies all the criteria below:
% * Within the ego car's lane.
% * In front of the ego car.
% * Closest to the ego car.


% 1. The lane is defined using a parabolic model, where y=ax^2+bx+c. a is
%    equal to half the road curvature, b=0, and c is the offset of the lane
%    boundaries relative to the ego car. Overall lane width is assumed to
%    be 3.6m, typical highway lane width.
laneWidth = 3.6;

% 2. The ego car is assumed to be traveling in the middle of its lane, with
%    1.8m on each side of it. So, c=+1.8m for the left lane boundary and
%    -1.8m for the right lane boundary.
halfLaneWidth = laneWidth/2;

maxX = cast(500.0,'double');
Selected = cast(-1,'int32');


if(width > 0)
    for i = 1:width
        type_obj = types(i);
        dis = range_bboxs(i);
        if type_obj == 3 || type_obj == 4
            dis = single(500.0);
        end
        del_height = dis * sin(elevation_angles(i));
        if abs(del_height) > 2
            dis = single(500.0);
        end
        speed = velocitys(i);
        angle = -azimuth_angles(i);
        yaw = 3.1415926/2 - headings(i);
        deltaYaw = yaw - EGOYAW;
        x = dis * cos(angle); % Longitudinal position of the track relative to ego
        y = dis * sin(angle); % Lateral position of the track relative to ego
        if dis < maxX && dis > 0
            yleftLane  = polyval([0, 0,  halfLaneWidth],x); % Half a lane to the left
            yrightLane = polyval([0, 0, -halfLaneWidth],x); % Half a lane to the right

            % Find a new lead car
            if(yrightLane <= y) && (y<=yleftLane)
                maxX = cast(dis,'double');
                Selected = i;
            end
        end
    end
end

if(Selected ~= -1)
    RelatedDistance = cast(range_bboxs(Selected),'double');
    yaw = 3.1415926/2 - headings(Selected);
    speed = velocitys(Selected);
    deltaYaw = yaw - EGOYAW;
    Vxx = speed * cos(deltaYaw);
    %Vyy = speed * sin(deltaYaw);
    RelatedSpeed = cast(-EGOV + Vxx,'double');
else
    RelatedDistance = 500;
    RelatedSpeed = 0.1;
end
